simulink model "s0212d"  (Simulink 6.3)
settings: Solver=ode45  SolverMode=SingleTasking  StartTime=0.0  StopTime=3  MaxStep=.01  RelTol=1e-3  AbsTol=1e-6
values from neighbouring files (symbols this model uses):
  cR = 0.05    [m0212d.m]    (also in m0218a.m; m0218e.m; m0251.m; m0252.m)
  g = 9.81    [m0208.m]    (also in m0212d.m; m0218a.m; m0218e.m; m0220b.m)
  l = l*1e-2    (= 0.1)    [m0212d.m]    (also in m0218a.m; m0218e.m; m0251.m = 0.2; m0252.m = 0.2)
  m = 0.5    [m0212d.m]    (also in m0218a.m; m0218e.m; m0251.m; m0252.m)
  omdach = 12    [m0212d.m]
  rP = rP*1e-2    (= 0.01)    [m0212d.m]    (also in m0218a.m; m0218e.m)
settings Model: LastModifiedBy=Froriep  StrictBusMsg=None
settings DataIOCC: LimitDataPoints=off  SaveOutput=off  TimeSaveName=t  SignalLoggingName=sigsOut
settings OptimizationCC: BooleanDataType=off  InlineInvariantSignals=on
settings DebuggingCC: SolverPrmCheckMsg=none
settings HardwareCC: TargetUnknown=on
settings GRTTargetCC: ModelReferenceCompliant=off  MatFileLogging=off

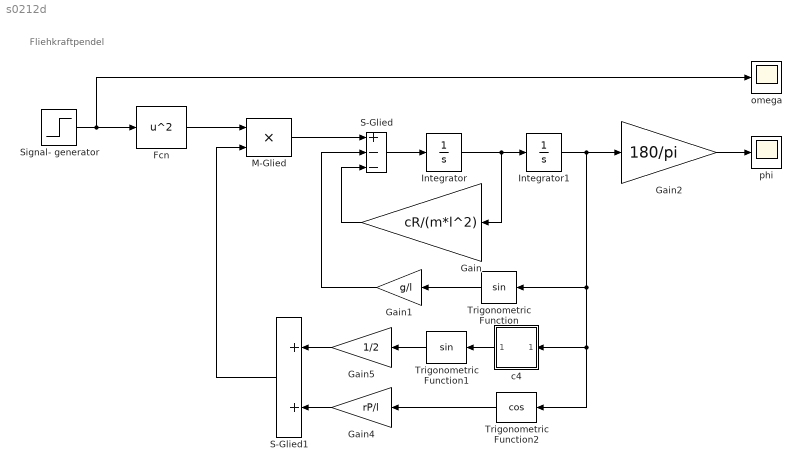
== system s0212d ==
  note: Fliehkraftpendel
  Fcn : Fcn  Expr=u^2
  Gain : Gain  Orientation=left  Gain=cR/(m*l^2)
  Gain1 : Gain  Orientation=left  Gain=g/l
  Gain2 : Gain  Gain=180/pi
  Gain4 : Gain  Orientation=left  Gain=rP/l
  Gain5 : Gain  Orientation=left  Gain=1/2
  Integrator : Integrator
  Integrator1 : Integrator
  M-Glied : Product  SaturateOnIntegerOverflow=on  InputSameDT=on
  S-Glied : Sum  Inputs=+--  SaturateOnIntegerOverflow=on  InputSameDT=on
  S-Glied1 : Sum  Orientation=left  SaturateOnIntegerOverflow=on  InputSameDT=on
  Signal- generator : Step  Time=.5  After=omdach  SampleTime=0  ZeroCross=off
  Trigonometric Function : Trigonometry  Orientation=left
  Trigonometric Function1 : Trigonometry  Orientation=left
  Trigonometric Function2 : Trigonometry  Orientation=left  Operator=cos
  c4 : Subsystem  Orientation=left  mask(P-Glied){@1=2}
      mask prompts: @1 "Beiwert"
      mask help: P-Glied
      mask init:
      | Kp=@1;
      mask Display: disp('2')
  omega : Scope
      settings: YMin=-1  YMax=20
  phi : Scope
      settings: YMax=100
  wires:
  S-Glied/1 -> Integrator/1
  M-Glied/1 -> S-Glied/1
  Fcn/1 -> M-Glied/1
  Integrator/1 -> Gain/1, Integrator1/1
  Gain/1 -> S-Glied/3
  Gain1/1 -> S-Glied/2
  Trigonometric Function/1 -> Gain1/1
  c4/1(Out1) -> Trigonometric Function1/1
  Signal- generator/1 -> Fcn/1, omega/1
  Integrator1/1 -> Trigonometric Function/1, c4/1(In1), Trigonometric Function2/1, Gain2/1
  Gain2/1 -> phi/1
  Trigonometric Function2/1 -> Gain4/1
  Trigonometric Function1/1 -> Gain5/1
  Gain5/1 -> S-Glied1/1
  Gain4/1 -> S-Glied1/2
  S-Glied1/1 -> M-Glied/2

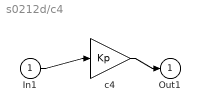
== system s0212d/c4 ==
  In1 : Inport
  c4 : Gain  Gain=Kp  SaturateOnIntegerOverflow=on
  Out1 : Outport
  wires:
  In1/1 -> c4/1
  c4/1 -> Out1/1
